simulink model "example_House_Ideal"  (R2018b)
settings: Solver=ode113  StartTime=0.0  StopTime=365*24*3600  RelTol=1e-3  EnableMultiTasking=on
undefined symbols (not defined in the file): path_carnot
libraries: carnot x7
settings Model: Creator=drhf  LastModifiedBy=drhf
settings DataIOCC: LimitDataPoints=on  SaveFormat=Array
settings OptimizationCC: ExpressionDepthLimit=2147483647  LifeSpan=inf
settings DebuggingCC: UnderspecifiedInitializationDetection=Classic  MergeDetectMultiDrivingBlocksExec=none  SolverPrmCheckMsg=warning  StateNameClashWarn=warning  SFUnexpectedBacktrackingDiag=warning  SFNoUnconditionalDefaultTransitionDiag=warning  SFExecutionAtInitializationDiag=none
settings HardwareCC: ProdBitPerPointer=32  ProdBitPerSizeT=32  ProdBitPerPtrDiffT=32  ProdLargestAtomicFloat=None  ProdIntDivRoundTo=Undefined  ProdEndianess=Unspecified  ProdWordSize=32  ProdHWDeviceType=32-bit Generic
settings ModelReferenceCC: PropagateSignalLabelsOutOfModel=off
settings SFSimCC: SimUseLocalCustomCode=off
settings RTWCC: RTWUseLocalCustomCode=off
settings CodeAppCC: StateflowObjectComments=on
settings GRTTargetCC: TargetLangStandard=C89/C90 (ANSI)  GeneratePreprocessorConditionals=Disable all  CombineOutputUpdateFcns=off  GRTInterface=on
settings ConfigComp: CovMetricSettings=dw  CovHtmlReporting=on  CovSaveCumulativeToWorkspaceVar=on  CovSaveSingleToWorkspaceVar=on  CovExternalEMLEnable=off

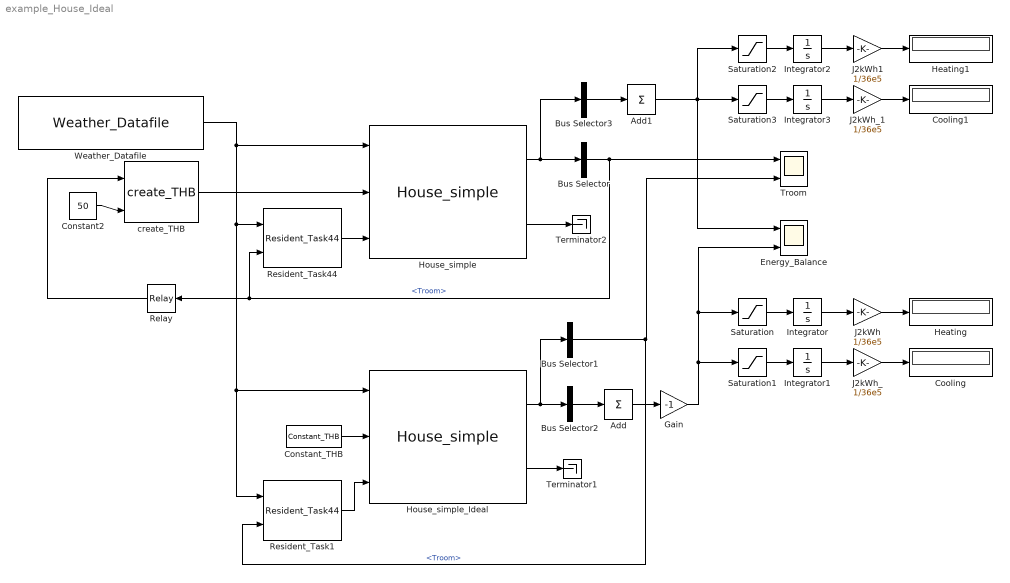
== system example_House_Ideal ==
  Add : Sum  Inputs=1
  Add1 : Sum  Inputs=1
  Bus Selector : BusSelector  OutputSignals=Troom
  Bus Selector1 : BusSelector  OutputSignals=Troom
  Bus Selector2 : BusSelector  OutputSignals=Qdot.Qdot_trans_wall,Qdot.Qdot_vent,Qdot.Qdot_ground,Qdot.Qdot_neighbour,Qdot.Qdot_internal,Qdot.Qdot_trans_window,Qdot.Qdot_solar  OutputAsBus=on
  Bus Selector3 : BusSelector  OutputSignals=Qdot.Qdot_h  OutputAsBus=on
  Constant2 : Constant  Value=50
  Constant_THB : carnot/Source/Simple/Constant_THB  t=20  mdot=0  p=1e5  mID=No Pressure Drop  fluid=Water  mix=0  mix2=0  mix3=0  dia=0.02  hgt=0
  Cooling : Display
  Cooling1 : Display
  Energy_Balance : Scope  NumInputPorts=2
  Gain : Gain  Gain=-1
  Heating : Display
  Heating1 : Display
  House_simple : carnot/Load/Houses/House_simple  tini=20  dtroom=inf  Tmeaninside=23.8  deltathetai=3.8  Tmeanoutside=11  deltathetae=9.3  tshift=319*3600  PathName=fullfile(path_carnot('libsl'), 'Load', 'Houses', 'House_simple', 'parameter_set')  FileName='SFH15_HouseSimple.mat'  userPath=off  userParam=off  Ahabit=140  Hroom=2.6  slabwidth=10  slablength=7  dwall=0.4  UAwall=0.162*(54.6+26.4)+0.182*((45.7+56.0)*2 -(12+4+3+4))  capa=500000  utot=0.1  gammat=0  cond_ground=2  cp_ground=800  rho_ground=2500  Awindow=[12 4 3 4]  AziWin=[0 90 -180 -90]  Uwindow="[1    1   1    1]*1.0"  Gwindow="[1    1   1    1]*0.585*(1-0.15)"  alpha=10  H=1.2  W=1  Nwin=4  Ventilationrate=0.4  Heatrecovery=0.6  pnom=1792  dtnom=15  expo=1.1  mcap=40000000  lin=10  qua=100
  House_simple_Ideal : carnot/Load/Houses/House_simple  tini=20  dtroom=0  Tmeaninside=23.8  deltathetai=3.8  Tmeanoutside=11  deltathetae=9.3  tshift=319*3600  PathName=fullfile(path_carnot('libsl'), 'Load', 'Houses', 'House_simple', 'parameter_set')  FileName='SFH15_HouseSimple.mat'  userPath=off  userParam=off  Ahabit=140  Hroom=2.6  slabwidth=10  slablength=7  dwall=0.4  UAwall=0.162*(54.6+26.4)+0.182*((45.7+56.0)*2 -(12+4+3+4))  capa=500000  utot=0.1  gammat=0  cond_ground=2  cp_ground=800  rho_ground=2500  Awindow=[12 4 3 4]  AziWin=[0 90 -180 -90]  Uwindow="[1    1   1    1]*1.0"  Gwindow="[1    1   1    1]*0.585*(1-0.15)"  alpha=10  H=1.2  W=1  Nwin=4  Ventilationrate=0.4  Heatrecovery=0.6  pnom=1792  dtnom=15  expo=1.1  mcap=40000000  lin=10  qua=100
  Integrator{,1..3} (4 alike) : Integrator
  J2kWh : Gain  Gain=1/36e5
  J2kWh1 : Gain  Gain=1/36e5
  J2kWh_ : Gain  Gain=1/36e5
  J2kWh_1 : Gain  Gain=1/36e5
  Relay : Relay  OnSwitchValue=20.1  OffSwitchValue=19.9  OnOutputValue=0  OffOutputValue=800/3600
  Resident_Task1 : carnot/Load/Houses/Resident_Task44  period=24*3600  rep_seq_te=[0 1 6 7 8 9 11 12 13 18 19 20 22 23]*3600  rep_seq_de=[1 5 1 1 1 2 1 1 4 2 1 2 1 1]*3600  rep_seq_ye=[105 55 392.5 457.5 420 55 250 55 120 170 615 420 442.5 355]  rep_seq_to=[0 6 7 8 9 11 12 13 14 15 17 18 20 21 22]*3600  rep_seq_do=[6 1 1 1 2 1 1 1 1 2 1 2 1 1 2]*3600  rep_seq_yo=[4 2 3 2 0 1 3 2 1 0 1 2 4 3 4]*60  Topen=24  Tclose=23  TrAboveTa=2  TaTooCold=12  timeFIR=24  TaIni=12  starttime=8  stoptime=22  TroomShadeOn=23.8  TroomShadeOff=22.8  SolarShadeOn=300  SolarShadeOff=200  max_shade=1  CalcAirComp=off  mdotCO2=0  mdotH2O=0  mdotVOC=0
  Resident_Task44 : carnot/Load/Houses/Resident_Task44  period=24*3600  rep_seq_te=[0 1 6 7 8 9 11 12 13 18 19 20 22 23]*3600  rep_seq_de=[1 5 1 1 1 2 1 1 4 2 1 2 1 1]*3600  rep_seq_ye=[105 55 392.5 457.5 420 55 250 55 120 170 615 420 442.5 355]  rep_seq_to=[0 6 7 8 9 11 12 13 14 15 17 18 20 21 22]*3600  rep_seq_do=[6 1 1 1 2 1 1 1 1 2 1 2 1 1 2]*3600  rep_seq_yo=[4 2 3 2 0 1 3 2 1 0 1 2 4 3 4]*60  Topen=24  Tclose=23  TrAboveTa=2  TaTooCold=12  timeFIR=24  TaIni=12  starttime=8  stoptime=22  TroomShadeOn=23.8  TroomShadeOff=22.8  SolarShadeOn=300  SolarShadeOff=200  max_shade=1  CalcAirComp=off  mdotCO2=0  mdotH2O=0  mdotVOC=0
  Saturation : Saturate  UpperLimit=inf  LowerLimit=0
  Saturation1 : Saturate  UpperLimit=0  LowerLimit=-inf
  Saturation2 : Saturate  UpperLimit=inf  LowerLimit=0
  Saturation3 : Saturate  UpperLimit=0  LowerLimit=-inf
  Terminator1 : Terminator
  Terminator2 : Terminator
  Troom : Scope  NumInputPorts=2
  Weather_Datafile : carnot/Weather/Weather_Datafile  PathName=path_carnot('data')  FileName='DE_TRY2010_04_averageYear.mat'  UserParam=off  VariableName=DE_TRY2010_04_averageYear  SampleTime=3600
  create_THB : carnot/Source/Simple/create_THB  p=1e5  fluid=Water  mix=0  mix2=0  mix3=0  dia=0.02  hgt=0  mID=No Pressure Drop
  wires:
  Weather_Datafile/1 -> Resident_Task1/1, House_simple_Ideal/1, Resident_Task44/1, House_simple/1
  create_THB/1 -> House_simple/2
  House_simple/1 -> Bus Selector/1, Bus Selector3/1
  House_simple/2 -> Terminator2/1
  Bus Selector/1 -> Troom/1, Resident_Task44/2, Relay/1  "<Troom>"
  House_simple_Ideal/2 -> Terminator1/1
  Bus Selector2/1 -> Add/1
  House_simple_Ideal/1 -> Bus Selector1/1, Bus Selector2/1
  Add/1 -> Gain/1
  Saturation/1 -> Integrator/1
  Integrator/1 -> J2kWh/1
  Saturation1/1 -> Integrator1/1
  Integrator1/1 -> J2kWh_/1
  J2kWh/1 -> Heating/1
  J2kWh_/1 -> Cooling/1
  Bus Selector1/1 -> Resident_Task1/2, Troom/2  "<Troom>"
  Bus Selector3/1 -> Add1/1
  Add1/1 -> Saturation2/1, Saturation3/1, Energy_Balance/1
  Saturation2/1 -> Integrator2/1
  Integrator2/1 -> J2kWh1/1
  Saturation3/1 -> Integrator3/1
  Integrator3/1 -> J2kWh_1/1
  J2kWh1/1 -> Heating1/1
  J2kWh_1/1 -> Cooling1/1
  Constant2/1 -> create_THB/2
  Gain/1 -> Saturation1/1, Energy_Balance/2, Saturation/1
  Resident_Task44/1 -> House_simple/3
  Relay/1 -> create_THB/1
  Constant_THB/1 -> House_simple_Ideal/2
  Resident_Task1/1 -> House_simple_Ideal/3
